simulink model "switch_operation"  (R2021a)
settings: Solver=VariableStepAuto  StartTime=0.0  StopTime=10.0  RelTol=1e-3
settings Model: Creator=DELL  LastModifiedBy=DELL

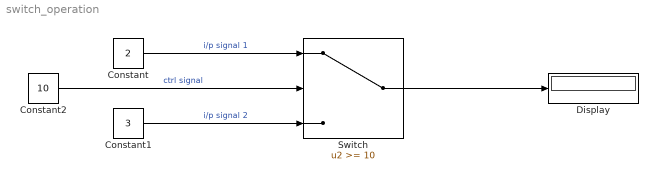
== system switch_operation ==
  Constant : Constant  Value=2
  Constant1 : Constant  Value=3
  Constant2 : Constant  Value=10
  Display : Display
  Switch : Switch  Threshold=10
  wires:
  Constant/1 -> Switch/1  "i/p signal 1"
  Constant1/1 -> Switch/3  "i/p signal 2"
  Constant2/1 -> Switch/2  "ctrl signal"
  Switch/1 -> Display/1
